simulink model "B20_ATMD_constrained_FDI"  (R2020b)
settings: Solver=ode45  StartTime=0.0  StopTime=tend  FixedStep=Ts  MaxStep=Ts  MinStep=0.005  RelTol=1e-2
values from neighbouring files (symbols this model uses):
  cstop = 5e7    (= 50000000)    [B20_AMD_main.m]    (also in B20_ATMD_main.m)
  EI = (1-FDIon)*EI    (= 0.4)    [B20_AMD_main.m]    (also in B20_ATMD_main.m)
  FDI_amp = FDIon*1*1000e5    (= 0)    [B20_AMD_main.m]    (also in B20_ATMD_main.m = 2000000)
  FDI_fr = 0.284687    [B20_AMD_main.m]    (also in B20_ATMD_main.m = 0.278681)
  FDIon = 0    [B20_AMD_main.m]    (also in B20_ATMD_main.m)
  K_lqr = lqr(A,B,Q,R)    [B20_AMD_main.m]    (also in B20_ATMD_main.m = 0*K_lqr)
  kstop = 4e6    (= 4000000)    [B20_AMD_main.m]    (also in B20_ATMD_main.m)
  Max_AMD_Disp = 0.5    [B20_AMD_main.m]    (also in B20_ATMD_main.m)
  MaxF = 2000e3    (= 2000000)    [B20_AMD_main.m]    (also in B20_ATMD_main.m)
  n_amd = n+1    (= 21)    [B20_AMD_main.m]    (also in B20_ATMD_main.m)
  Sys_con = ss(A,[E B],C,D)    [B20_AMD_main.m]    (also in B20_ATMD_main.m)
  Sys_unc = ss(A_ref,E_ref,C_ref,DD_ref)    [B20_AMD_main.m]    (also in B20_ATMD_main.m)
libraries: dspindex x2
settings Model: Creator=drsoto  LastModifiedBy=ferch
settings SolverCC: AlgebraicLoopSolver=LineSearch
settings DataIOCC: ReturnWorkspaceOutputs=off
settings DebuggingCC: AlgebraicLoopMsg=none  ArithmeticOperatorsInVariantConditions=warning
settings SFSimCC: SimUseLocalCustomCode=off  CustomCodeUndefinedFunction=UseInterfaceOnly
settings RTWCC: RTWUseLocalCustomCode=off
settings CodeAppCC: StateflowObjectComments=on

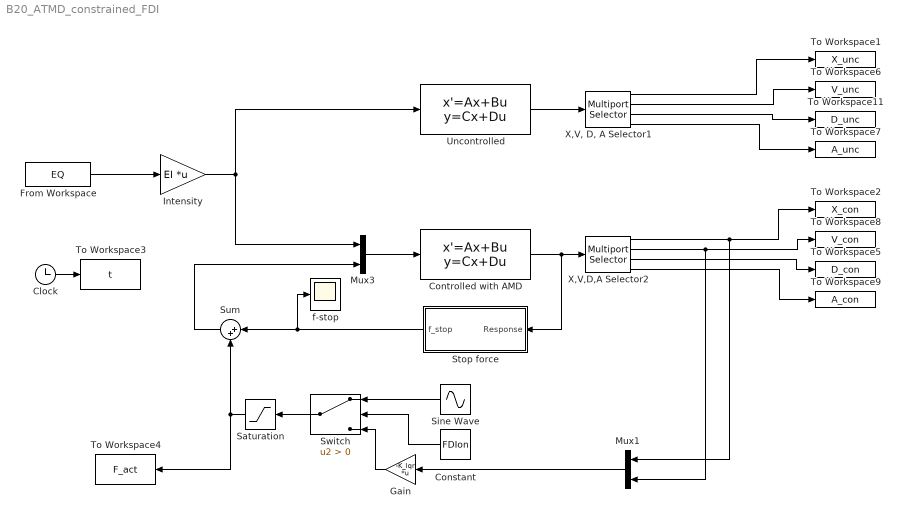
== system B20_ATMD_constrained_FDI ==
  Clock : Clock
  Constant : Constant  Value=FDIon
  Controlled with AMD : StateSpace  A=Sys_con.A  B=Sys_con.B  C=Sys_con.C  D=Sys_con.D  InitialCondition=0
  From Workspace : FromWorkspace  VariableName=EQ  SampleTime=-1
  Gain : Gain  Gain=-K_lqr  Multiplication=Matrix(K*u)
  Intensity : Gain  Gain=EI  Multiplication=Matrix(K*u)
  Mux1 : Mux  Inputs=2
  Mux3 : Mux  Inputs=2
  Saturation : Saturate  UpperLimit=MaxF  LowerLimit=-MaxF
  Sine Wave : Sin  Amplitude=FDI_amp  Frequency=FDI_fr*2*pi  SampleTime=0
  Stop force : Subsystem
  Sum : Sum  Inputs=|++
  Switch : Switch  Criteria=u2 > Threshold
  To Workspace1 : ToWorkspace  VariableName=X_unc  SampleTime=-1
  To Workspace11 : ToWorkspace  VariableName=D_unc  SampleTime=-1
  To Workspace2 : ToWorkspace  VariableName=X_con  SampleTime=-1
  To Workspace3 : ToWorkspace  VariableName=t  SampleTime=-1
      settings: Save2DSignal=2-D array (concatenate along first dimension)
  To Workspace4 : ToWorkspace  VariableName=F_act  SampleTime=-1
  To Workspace5 : ToWorkspace  VariableName=D_con  SampleTime=-1
  To Workspace6 : ToWorkspace  VariableName=V_unc  SampleTime=-1
  To Workspace7 : ToWorkspace  VariableName=A_unc  SampleTime=-1
  To Workspace8 : ToWorkspace  VariableName=V_con  SampleTime=-1
  To Workspace9 : ToWorkspace  VariableName=A_con  SampleTime=-1
  Uncontrolled : StateSpace  A=Sys_unc.A  B=Sys_unc.B  C=Sys_unc.C  D=Sys_unc.D  InitialCondition=0
  "X,V, D, A Selector1" : dspindex/Multiport Selector  rowsOrCols=Rows  idxCellArray={ 1:n,n+1:2*n,2*n+1:3*n,3*n+1:4*n}  idxErrMode=Clip Index
  X,V,D,A Selector2 : dspindex/Multiport Selector  rowsOrCols=Rows  idxCellArray={ 1:n_amd,n_amd+1:2*n_amd,2*n_amd+1:3*n_amd,3*n_amd+1:4*n_amd}  idxErrMode=Clip Index
  f-stop : Scope
  wires:
  Intensity/1 -> Uncontrolled/1, Mux3/1
  Uncontrolled/1 -> "X,V, D, A Selector1"/1
  From Workspace/1 -> Intensity/1
  Controlled with AMD/1 -> Stop force/1(Response), X,V,D,A Selector2/1
  Mux1/1 -> Gain/1
  Clock/1 -> To Workspace3/1
  "X,V, D, A Selector1"/2 -> To Workspace6/1
  Mux3/1 -> Controlled with AMD/1
  "X,V, D, A Selector1"/4 -> To Workspace7/1
  "X,V, D, A Selector1"/3 -> To Workspace11/1
  X,V,D,A Selector2/3 -> To Workspace5/1
  X,V,D,A Selector2/4 -> To Workspace9/1
  "X,V, D, A Selector1"/1 -> To Workspace1/1
  X,V,D,A Selector2/1 -> Mux1/1, To Workspace2/1
  X,V,D,A Selector2/2 -> To Workspace8/1, Mux1/2
  Switch/1 -> Saturation/1
  Constant/1 -> Switch/2
  Gain/1 -> Switch/3
  Sine Wave/1 -> Switch/1
  Stop force/1(f_stop) -> f-stop/1, Sum/1
  Saturation/1 -> To Workspace4/1, Sum/2
  Sum/1 -> Mux3/2

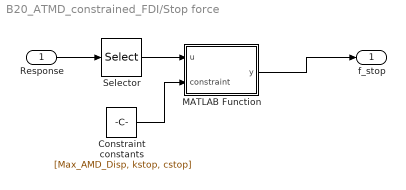
== system B20_ATMD_constrained_FDI/Stop force ==
  Response : Inport
  Constraint constants : Constant  Value=[Max_AMD_Disp, kstop, cstop]
  MATLAB Function : MATLAB Function  TreatAsAtomicUnit=on
  Selector : Selector  InputPortWidth=4*n_amd  IndexOptions=Index vector (dialog)  Indices=[n_amd 2*n_amd 4*n_amd]  OutputSizes=1
  f_stop : Outport
  wires:
  Selector/1 -> MATLAB Function/1(u)
  Response/1 -> Selector/1
  MATLAB Function/1(y) -> f_stop/1
  Constraint constants/1 -> MATLAB Function/2(constraint)

== matlab function B20_ATMD_constrained_FDI/Stop force/MATLAB Function ==
  data: u input; y output; constraint input
function y = fcn(u, constraint)

x = u(1);
v = u(2);
kstop=constraint(2);
cstop=constraint(3);
lim = constraint(1);

if (x > lim && v<=0) || (x < -lim && v>=0)
    fstop = kstop*x;
elseif (x > lim && v>0) || (x < -lim && v<0)
    fstop = kstop*x+cstop*v;
else 
    fstop = 0;
end
y = -fstop;
